simulink model "Gesamt"  (R2015b)
settings: Solver=ode3  SolverMode=SingleTasking  StartTime=0.0  StopTime=inf  RelTol=1e-3
InitFcn:
  | Reglerauslegung
values from neighbouring files (symbols this model uses):
  aMax = 498    [Reglerauslegung.m]
  aMaxPsi = 1    [Reglerauslegung.m]
  Blindzeit = 25    [Reglerauslegung.m]
  dt = 0.005    [Reglerauslegung.m]
  K1 = place(AI1,BI1,pWunschI1)    [Reglerauslegung.m]
  K2 = place(A2,B2,pWunsch2)    [Reglerauslegung.m]
  K3 = place(A3,B3,pWunsch3)    [Reglerauslegung.m]
  Kx = 0.9575    [Reglerauslegung.m]
  Ky = 0.9575    [Reglerauslegung.m]
  Tx = 1/4.1668    (= 0.239992320246)    [Reglerauslegung.m]
  Ty = 1/4.1668    (= 0.239992320246)    [Reglerauslegung.m]
  vMax = 403    [Reglerauslegung.m]
  vMaxPsi = 3    [Reglerauslegung.m]
undefined symbols (not defined in the file or in its folder): sigbuilder_block
libraries: simulink x5, xpcutilitieslib x1
(part 3 of 3)

== matlab function Gesamt/Regelung1/Zustandsregler/Winkelentstoerung ==
  data: Ist input; Soll input; Out output



function Out = Winkel(Ist,Soll)

Ist = mod(Ist, 2*pi);      % Normierung des Ist-Winkels auf das Intervall 0° - 360°
Soll = mod(Soll, 2*pi);    % Normierung des Soll-Winkels auf das Intervall 0° - 360°

if (abs(Soll-Ist) <= pi)   % (1)
    
    Out = Soll - Ist;      % (2)
    
else
    
     if (Soll > Ist)                % (3)
        Out = Soll - Ist - 2*pi;    % (4)
     else
         Out = Soll - Ist + 2*pi;   % (5)
     end
end

% Problem: 
% Beim Durchschreiten der Grenze 0°/360° entsteht ein Sprung in
% der Regeldifferenz beim Winkel, der zu einer unkontrollierten Rotation
% des Robotino führt
% 
% Lösung: 
% Impelementierung einer Fallunterscheidung, die die tatsächliche
% Regeldifferenz unter Berücksichtigung der Grenze 0°/360° ausgibt
% 
% Ansatz: 
% Prüfung, ob die vorgegebene Trajektorie über die kritische Grenze
% führt (1). Führt die Trajektorie über die kritische Grenze, ist
% der Betrag der Differenz zwischen Soll- und Istwert > pi.
% 
% Bei unkritischen Trajektorien wird die Regeldifferenz über die Formel (2)
% zurückgegeben.
%
% Bei kritischen Trajektorien muss zuerst unterschieden werden, in welchem
% Drehsinn die kritische Grenze durchschritten wird (3). Bei positivem
% Drehsinn wird die Differenz nach Formel (4) ermittelt, bei negativem
% Drehsinn wird die Differenz nach Formal (5) ermittelt. 
%
% Die Ausgabe der Regeldifferenz erfolgt immer in Richtung und Betrag, bei
% einem positiven Vorzeichen befindet sich die Sollposition in mathematisch
% positivem Drehsinn, bei einem negativen Vorzeichen befindet sie sich in
% mathematisch negativem Drehsinn. Der Betrag gibt die verbleibene
% Winkeldifferenz zur Sollposition an.

== matlab function Gesamt/Regelung1/enable  ==
  data: BereichsModus input; enableBereich input; enableKamera input; enableBeobachter input; enable output; enableKoord input; enableFlogik input
function enable  = enable(BereichsModus, enableBereich,enableKamera,enableBeobachter,enableKoord,enableFlogik)
    if BereichsModus == 1
        % Fertigungsbereich
        if enableBereich && (enableKamera || enableKoord )&& enableBeobachter && enableFlogik
            enable = 1;
        else 
            enable = 0;
        end
    else
        % Transportbereich
        if enableKamera || enableKoord 
            % mindestens kamera oder beobachter muessen funktionieren            
            enable = 1;
        else
            % sonst nix fahren 
            enable = 0;
        end
    end
    
end

== matlab function Gesamt/Regelung1/u(x,v)  ==
  data: v1 input; v2 input; v3 input; x1 input; x2 input; x3 input; x4 input; u1 output; u2 output; u3 output; Tx parameter; Ty parameter; Kx parameter; Ky parameter
function [u1, u2, u3]= inputLinearisierung(v1,v2,v3,x1,x2,x3,x4,Tx,Ty,Kx,Ky)


%u1 = (Ty*x1 - Tx*x1 + Ty*v1*cos(x4) + Tx*v2*sin(x4) + Tx*x1*cos(x4)^2 - Ty*x1*cos(x4)^2 - (Tx*x2*sin(2*x4))/2 + (Ty*x2*sin(2*x4))/2 + Tx*Ty*x2*x3)/Ty;
%u2 = -(Ty*x2 - Tx*x2 - Tx*v2*cos(x4) + Ty*v1*sin(x4) + Tx*x2*cos(x4)^2 - Ty*x2*cos(x4)^2 + (Tx*x1*sin(2*x4))/2 - (Ty*x1*sin(2*x4))/2 + Tx*Ty*x1*x3)/Tx;
u1 = (Ty*x1 - Tx*x1 + Tx*x1*cos(x4)^2 - Ty*x1*cos(x4)^2 - (Tx*x2*sin(2*x4))/2 + (Ty*x2*sin(2*x4))/2 + Kx*Ty*v1*cos(x4) + Ky*Tx*v2*sin(x4) + Tx*Ty*x2*x3)/(Kx*Ty);
u2 = -(Ty*x2 - Tx*x2 + Tx*x2*cos(x4)^2 - Ty*x2*cos(x4)^2 + (Tx*x1*sin(2*x4))/2 - (Ty*x1*sin(2*x4))/2 - Ky*Tx*v2*cos(x4) + Kx*Ty*v1*sin(x4) + Tx*Ty*x1*x3)/(Ky*Tx);
u3 = v3;

== matlab function Gesamt/Regelung1/z(x) ==
  data: x1 input; x2 input; x3 input; x4 input; z1 output; z5 output; z2 output; z6 output; x5 input; x6 input; z3 output; z4 output
function [z1,z5,z2,z6,z3,z4]= zustandsTrafo(x1,x2,x3,x4,x5,x6)

z1 = cos(x4) * x1 - sin(x4) * x2;
z2 = sin(x4) * x1 + cos(x4) * x2;
z3 = x3;
z4 = x4;
z5 = x5;
z6 = x6;
